simulink model "c960x4096_x14_7_r2013b_frb"  (R2013b)
settings: Solver=ode45  StartTime=0.0  StopTime=40960  RelTol=1e-3
undefined symbols (not defined in the file): sfp
libraries: xbsIndex_r4 x14620, casper_library_misc x61, dspsigops x32, casper_library_multipliers x24, simulink x18, xps_library x18
(part 11 of 79)

== system c960x4096_x14_7_r2013b_frb/p0_scale/SCALE_Re_&_Im_2 ==
  P_S : Inport
  SCALE : Inport  Port=2
  Convert : xbsIndex_r4/Convert  gui_display_data_type=Fixed-point  arith_type="Signed  (2's comp)"  n_bits=8  bin_pt=5  float_type=Single  exp_bits=8  fraction_bits=24  quantization=Truncate  overflow=Wrap  en=off  latency=0  dbl_ovrd=off  pipeline=off  block_type=convert
  Convert1 : xbsIndex_r4/Convert  gui_display_data_type=Fixed-point  arith_type="Signed  (2's comp)"  n_bits=8  bin_pt=5  float_type=Single  exp_bits=8  fraction_bits=24  quantization=Truncate  overflow=Wrap  en=off  latency=0  dbl_ovrd=off  pipeline=off  block_type=convert
  Mult : xbsIndex_r4/Mult  precision=Full  arith_type="Signed  (2's comp)"  n_bits=16  bin_pt=14  quantization=Truncate  overflow=Wrap  en=off  latency=4  dbl_ovrd=off  use_behavioral_HDL=off  opt=Speed  use_embedded=on  optimum_pipeline=off  pipeline=on  use_rpm=on  placement_style=Triangular  block_type=mult
  Mult1 : xbsIndex_r4/Mult  precision=Full  arith_type="Signed  (2's comp)"  n_bits=16  bin_pt=14  quantization=Truncate  overflow=Wrap  en=off  latency=4  dbl_ovrd=off  use_behavioral_HDL=off  opt=Speed  use_embedded=on  optimum_pipeline=off  pipeline=on  use_rpm=on  placement_style=Triangular  block_type=mult
  Reinterpret : xbsIndex_r4/Reinterpret  force_arith_type=on  arith_type="Signed  (2's comp)"  force_bin_pt=on  bin_pt=17  block_type=reinterpret
  Reinterpret1 : xbsIndex_r4/Reinterpret  force_arith_type=on  arith_type="Signed  (2's comp)"  force_bin_pt=on  bin_pt=17  block_type=reinterpret
  Slice : xbsIndex_r4/Slice  nbits=18  boolean_output=off  mode=Upper Bit Location + Width  bit1=0  base1=MSB of Input  bit0=0  base0=LSB of Input  dbl_ovrd=off  block_type=slice
  Slice1 : xbsIndex_r4/Slice  nbits=18  boolean_output=off  mode=Lower Bit Location + Width  bit1=0  base1=MSB of Input  bit0=0  base0=LSB of Input  dbl_ovrd=off  block_type=slice
  Re : Outport
  Im : Outport  Port=2
  wires:
  SCALE/1 -> Mult/2, Mult1/2
  P_S/1 -> Slice1/1, Slice/1
  Convert1/1 -> Im/1
  Convert/1 -> Re/1
  Mult1/1 -> Convert1/1
  Mult/1 -> Convert/1
  Reinterpret/1 -> Mult1/1
  Reinterpret1/1 -> Mult/1
  Slice1/1 -> Reinterpret/1
  Slice/1 -> Reinterpret1/1

== system c960x4096_x14_7_r2013b_frb/p0_scale/SCALE_Re_&_Im_3 ==
  P_S : Inport
  SCALE : Inport  Port=2
  Convert : xbsIndex_r4/Convert  gui_display_data_type=Fixed-point  arith_type="Signed  (2's comp)"  n_bits=8  bin_pt=5  float_type=Single  exp_bits=8  fraction_bits=24  quantization=Truncate  overflow=Wrap  en=off  latency=0  dbl_ovrd=off  pipeline=off  block_type=convert
  Convert1 : xbsIndex_r4/Convert  gui_display_data_type=Fixed-point  arith_type="Signed  (2's comp)"  n_bits=8  bin_pt=5  float_type=Single  exp_bits=8  fraction_bits=24  quantization=Truncate  overflow=Wrap  en=off  latency=0  dbl_ovrd=off  pipeline=off  block_type=convert
  Mult : xbsIndex_r4/Mult  precision=Full  arith_type="Signed  (2's comp)"  n_bits=16  bin_pt=14  quantization=Truncate  overflow=Wrap  en=off  latency=4  dbl_ovrd=off  use_behavioral_HDL=off  opt=Speed  use_embedded=on  optimum_pipeline=off  pipeline=on  use_rpm=on  placement_style=Triangular  block_type=mult
  Mult1 : xbsIndex_r4/Mult  precision=Full  arith_type="Signed  (2's comp)"  n_bits=16  bin_pt=14  quantization=Truncate  overflow=Wrap  en=off  latency=4  dbl_ovrd=off  use_behavioral_HDL=off  opt=Speed  use_embedded=on  optimum_pipeline=off  pipeline=on  use_rpm=on  placement_style=Triangular  block_type=mult
  Reinterpret : xbsIndex_r4/Reinterpret  force_arith_type=on  arith_type="Signed  (2's comp)"  force_bin_pt=on  bin_pt=17  block_type=reinterpret
  Reinterpret1 : xbsIndex_r4/Reinterpret  force_arith_type=on  arith_type="Signed  (2's comp)"  force_bin_pt=on  bin_pt=17  block_type=reinterpret
  Slice : xbsIndex_r4/Slice  nbits=18  boolean_output=off  mode=Upper Bit Location + Width  bit1=0  base1=MSB of Input  bit0=0  base0=LSB of Input  dbl_ovrd=off  block_type=slice
  Slice1 : xbsIndex_r4/Slice  nbits=18  boolean_output=off  mode=Lower Bit Location + Width  bit1=0  base1=MSB of Input  bit0=0  base0=LSB of Input  dbl_ovrd=off  block_type=slice
  Re : Outport
  Im : Outport  Port=2
  wires:
  SCALE/1 -> Mult/2, Mult1/2
  P_S/1 -> Slice1/1, Slice/1
  Convert1/1 -> Im/1
  Convert/1 -> Re/1
  Mult1/1 -> Convert1/1
  Mult/1 -> Convert/1
  Reinterpret/1 -> Mult1/1
  Reinterpret1/1 -> Mult/1
  Slice1/1 -> Reinterpret/1
  Slice/1 -> Reinterpret1/1

== system c960x4096_x14_7_r2013b_frb/p0_scale/SCALE_Re_&_Im_4 ==
  P_S : Inport
  SCALE : Inport  Port=2
  Convert : xbsIndex_r4/Convert  gui_display_data_type=Fixed-point  arith_type="Signed  (2's comp)"  n_bits=8  bin_pt=5  float_type=Single  exp_bits=8  fraction_bits=24  quantization=Truncate  overflow=Wrap  en=off  latency=0  dbl_ovrd=off  pipeline=off  block_type=convert
  Convert1 : xbsIndex_r4/Convert  gui_display_data_type=Fixed-point  arith_type="Signed  (2's comp)"  n_bits=8  bin_pt=5  float_type=Single  exp_bits=8  fraction_bits=24  quantization=Truncate  overflow=Wrap  en=off  latency=0  dbl_ovrd=off  pipeline=off  block_type=convert
  Mult : xbsIndex_r4/Mult  precision=Full  arith_type="Signed  (2's comp)"  n_bits=16  bin_pt=14  quantization=Truncate  overflow=Wrap  en=off  latency=4  dbl_ovrd=off  use_behavioral_HDL=off  opt=Speed  use_embedded=on  optimum_pipeline=off  pipeline=on  use_rpm=on  placement_style=Triangular  block_type=mult
  Mult1 : xbsIndex_r4/Mult  precision=Full  arith_type="Signed  (2's comp)"  n_bits=16  bin_pt=14  quantization=Truncate  overflow=Wrap  en=off  latency=4  dbl_ovrd=off  use_behavioral_HDL=off  opt=Speed  use_embedded=on  optimum_pipeline=off  pipeline=on  use_rpm=on  placement_style=Triangular  block_type=mult
  Reinterpret : xbsIndex_r4/Reinterpret  force_arith_type=on  arith_type="Signed  (2's comp)"  force_bin_pt=on  bin_pt=17  block_type=reinterpret
  Reinterpret1 : xbsIndex_r4/Reinterpret  force_arith_type=on  arith_type="Signed  (2's comp)"  force_bin_pt=on  bin_pt=17  block_type=reinterpret
  Slice : xbsIndex_r4/Slice  nbits=18  boolean_output=off  mode=Upper Bit Location + Width  bit1=0  base1=MSB of Input  bit0=0  base0=LSB of Input  dbl_ovrd=off  block_type=slice
  Slice1 : xbsIndex_r4/Slice  nbits=18  boolean_output=off  mode=Lower Bit Location + Width  bit1=0  base1=MSB of Input  bit0=0  base0=LSB of Input  dbl_ovrd=off  block_type=slice
  Re : Outport
  Im : Outport  Port=2
  wires:
  SCALE/1 -> Mult/2, Mult1/2
  P_S/1 -> Slice1/1, Slice/1
  Convert1/1 -> Im/1
  Convert/1 -> Re/1
  Mult1/1 -> Convert1/1
  Mult/1 -> Convert/1
  Reinterpret/1 -> Mult1/1
  Reinterpret1/1 -> Mult/1
  Slice1/1 -> Reinterpret/1
  Slice/1 -> Reinterpret1/1

== system c960x4096_x14_7_r2013b_frb/p0_scale/SCALE_Re_&_Im_5 ==
  P_S : Inport
  SCALE : Inport  Port=2
  Convert : xbsIndex_r4/Convert  gui_display_data_type=Fixed-point  arith_type="Signed  (2's comp)"  n_bits=8  bin_pt=5  float_type=Single  exp_bits=8  fraction_bits=24  quantization=Truncate  overflow=Wrap  en=off  latency=0  dbl_ovrd=off  pipeline=off  block_type=convert
  Convert1 : xbsIndex_r4/Convert  gui_display_data_type=Fixed-point  arith_type="Signed  (2's comp)"  n_bits=8  bin_pt=5  float_type=Single  exp_bits=8  fraction_bits=24  quantization=Truncate  overflow=Wrap  en=off  latency=0  dbl_ovrd=off  pipeline=off  block_type=convert
  Mult : xbsIndex_r4/Mult  precision=Full  arith_type="Signed  (2's comp)"  n_bits=16  bin_pt=14  quantization=Truncate  overflow=Wrap  en=off  latency=4  dbl_ovrd=off  use_behavioral_HDL=off  opt=Speed  use_embedded=on  optimum_pipeline=off  pipeline=on  use_rpm=on  placement_style=Triangular  block_type=mult
  Mult1 : xbsIndex_r4/Mult  precision=Full  arith_type="Signed  (2's comp)"  n_bits=16  bin_pt=14  quantization=Truncate  overflow=Wrap  en=off  latency=4  dbl_ovrd=off  use_behavioral_HDL=off  opt=Speed  use_embedded=on  optimum_pipeline=off  pipeline=on  use_rpm=on  placement_style=Triangular  block_type=mult
  Reinterpret : xbsIndex_r4/Reinterpret  force_arith_type=on  arith_type="Signed  (2's comp)"  force_bin_pt=on  bin_pt=17  block_type=reinterpret
  Reinterpret1 : xbsIndex_r4/Reinterpret  force_arith_type=on  arith_type="Signed  (2's comp)"  force_bin_pt=on  bin_pt=17  block_type=reinterpret
  Slice : xbsIndex_r4/Slice  nbits=18  boolean_output=off  mode=Upper Bit Location + Width  bit1=0  base1=MSB of Input  bit0=0  base0=LSB of Input  dbl_ovrd=off  block_type=slice
  Slice1 : xbsIndex_r4/Slice  nbits=18  boolean_output=off  mode=Lower Bit Location + Width  bit1=0  base1=MSB of Input  bit0=0  base0=LSB of Input  dbl_ovrd=off  block_type=slice
  Re : Outport
  Im : Outport  Port=2
  wires:
  SCALE/1 -> Mult/2, Mult1/2
  P_S/1 -> Slice1/1, Slice/1
  Convert1/1 -> Im/1
  Convert/1 -> Re/1
  Mult1/1 -> Convert1/1
  Mult/1 -> Convert/1
  Reinterpret/1 -> Mult1/1
  Reinterpret1/1 -> Mult/1
  Slice1/1 -> Reinterpret/1
  Slice/1 -> Reinterpret1/1

== system c960x4096_x14_7_r2013b_frb/p0_scale/SCALE_Re_&_Im_6 ==
  P_S : Inport
  SCALE : Inport  Port=2
  Convert : xbsIndex_r4/Convert  gui_display_data_type=Fixed-point  arith_type="Signed  (2's comp)"  n_bits=8  bin_pt=5  float_type=Single  exp_bits=8  fraction_bits=24  quantization=Truncate  overflow=Wrap  en=off  latency=0  dbl_ovrd=off  pipeline=off  block_type=convert
  Convert1 : xbsIndex_r4/Convert  gui_display_data_type=Fixed-point  arith_type="Signed  (2's comp)"  n_bits=8  bin_pt=5  float_type=Single  exp_bits=8  fraction_bits=24  quantization=Truncate  overflow=Wrap  en=off  latency=0  dbl_ovrd=off  pipeline=off  block_type=convert
  Mult : xbsIndex_r4/Mult  precision=Full  arith_type="Signed  (2's comp)"  n_bits=16  bin_pt=14  quantization=Truncate  overflow=Wrap  en=off  latency=4  dbl_ovrd=off  use_behavioral_HDL=off  opt=Speed  use_embedded=on  optimum_pipeline=off  pipeline=on  use_rpm=on  placement_style=Triangular  block_type=mult
  Mult1 : xbsIndex_r4/Mult  precision=Full  arith_type="Signed  (2's comp)"  n_bits=16  bin_pt=14  quantization=Truncate  overflow=Wrap  en=off  latency=4  dbl_ovrd=off  use_behavioral_HDL=off  opt=Speed  use_embedded=on  optimum_pipeline=off  pipeline=on  use_rpm=on  placement_style=Triangular  block_type=mult
  Reinterpret : xbsIndex_r4/Reinterpret  force_arith_type=on  arith_type="Signed  (2's comp)"  force_bin_pt=on  bin_pt=17  block_type=reinterpret
  Reinterpret1 : xbsIndex_r4/Reinterpret  force_arith_type=on  arith_type="Signed  (2's comp)"  force_bin_pt=on  bin_pt=17  block_type=reinterpret
  Slice : xbsIndex_r4/Slice  nbits=18  boolean_output=off  mode=Upper Bit Location + Width  bit1=0  base1=MSB of Input  bit0=0  base0=LSB of Input  dbl_ovrd=off  block_type=slice
  Slice1 : xbsIndex_r4/Slice  nbits=18  boolean_output=off  mode=Lower Bit Location + Width  bit1=0  base1=MSB of Input  bit0=0  base0=LSB of Input  dbl_ovrd=off  block_type=slice
  Re : Outport
  Im : Outport  Port=2
  wires:
  SCALE/1 -> Mult/2, Mult1/2
  P_S/1 -> Slice1/1, Slice/1
  Convert1/1 -> Im/1
  Convert/1 -> Re/1
  Mult1/1 -> Convert1/1
  Mult/1 -> Convert/1
  Reinterpret/1 -> Mult1/1
  Reinterpret1/1 -> Mult/1
  Slice1/1 -> Reinterpret/1
  Slice/1 -> Reinterpret1/1

== system c960x4096_x14_7_r2013b_frb/p0_scale/SCALE_Re_&_Im_7 ==
  P_S : Inport
  SCALE : Inport  Port=2
  Convert : xbsIndex_r4/Convert  gui_display_data_type=Fixed-point  arith_type="Signed  (2's comp)"  n_bits=8  bin_pt=5  float_type=Single  exp_bits=8  fraction_bits=24  quantization=Truncate  overflow=Wrap  en=off  latency=0  dbl_ovrd=off  pipeline=off  block_type=convert
  Convert1 : xbsIndex_r4/Convert  gui_display_data_type=Fixed-point  arith_type="Signed  (2's comp)"  n_bits=8  bin_pt=5  float_type=Single  exp_bits=8  fraction_bits=24  quantization=Truncate  overflow=Wrap  en=off  latency=0  dbl_ovrd=off  pipeline=off  block_type=convert
  Mult : xbsIndex_r4/Mult  precision=Full  arith_type="Signed  (2's comp)"  n_bits=16  bin_pt=14  quantization=Truncate  overflow=Wrap  en=off  latency=4  dbl_ovrd=off  use_behavioral_HDL=off  opt=Speed  use_embedded=on  optimum_pipeline=off  pipeline=on  use_rpm=on  placement_style=Triangular  block_type=mult
  Mult1 : xbsIndex_r4/Mult  precision=Full  arith_type="Signed  (2's comp)"  n_bits=16  bin_pt=14  quantization=Truncate  overflow=Wrap  en=off  latency=4  dbl_ovrd=off  use_behavioral_HDL=off  opt=Speed  use_embedded=on  optimum_pipeline=off  pipeline=on  use_rpm=on  placement_style=Triangular  block_type=mult
  Reinterpret : xbsIndex_r4/Reinterpret  force_arith_type=on  arith_type="Signed  (2's comp)"  force_bin_pt=on  bin_pt=17  block_type=reinterpret
  Reinterpret1 : xbsIndex_r4/Reinterpret  force_arith_type=on  arith_type="Signed  (2's comp)"  force_bin_pt=on  bin_pt=17  block_type=reinterpret
  Slice : xbsIndex_r4/Slice  nbits=18  boolean_output=off  mode=Upper Bit Location + Width  bit1=0  base1=MSB of Input  bit0=0  base0=LSB of Input  dbl_ovrd=off  block_type=slice
  Slice1 : xbsIndex_r4/Slice  nbits=18  boolean_output=off  mode=Lower Bit Location + Width  bit1=0  base1=MSB of Input  bit0=0  base0=LSB of Input  dbl_ovrd=off  block_type=slice
  Re : Outport
  Im : Outport  Port=2
  wires:
  SCALE/1 -> Mult/2, Mult1/2
  P_S/1 -> Slice1/1, Slice/1
  Convert1/1 -> Im/1
  Convert/1 -> Re/1
  Mult1/1 -> Convert1/1
  Mult/1 -> Convert/1
  Reinterpret/1 -> Mult1/1
  Reinterpret1/1 -> Mult/1
  Slice1/1 -> Reinterpret/1
  Slice/1 -> Reinterpret1/1

== system c960x4096_x14_7_r2013b_frb/p1_adc/Subsystem1 ==
  In1 : Inport
  In2 : Inport  Port=2
  In3 : Inport  Port=3
  In4 : Inport  Port=4
  In5 : Inport  Port=5
  In6 : Inport  Port=6
  In7 : Inport  Port=7
  In8 : Inport  Port=8
  In9 : Inport  Port=9
  In10 : Inport  Port=10
  In11 : Inport  Port=11
  In12 : Inport  Port=12
  In13 : Inport  Port=13
  In14 : Inport  Port=14
  In15 : Inport  Port=15
  In16 : Inport  Port=16
  Delay{1..10,18..20,22..24} (16 alike) : xbsIndex_r4/Delay  rst=off  infoeditControl=Selection of Reset will increase slice count due to use of real FFs and instead of SRLs  en=off  latency=1  dbl_ovrd=off  reg_retiming=on  block_type=delay
      settings: block_version=11.4
  DocBlock : simulink/Model-Wide Utilities/DocBlock  DocumentType=Text
      content=|
      | - JMR, 04/30/13
      | Converter blocks needed to convert the ASIAA ADC output from offset
      | notation (0 - 255 corresponds to -full scale to +full scale) to 2's
      | complement (-128 to +127).  Per email from Glenn Jones, 04/17/13
  bus_create : Subsystem  AncestorBlock=casper_library_flow_control/bus_create  mask(bus_create){inputNum=16}
      mask prompts: inputNum "Number of inputs:"
      mask init:
      | bus_create_init(gcb,...
      |     'inputNum', inputNum);
  converter : Subsystem
  converter1 : Subsystem
  converter10 : Subsystem
  converter11 : Subsystem
  converter12 : Subsystem
  converter13 : Subsystem
  converter14 : Subsystem
  converter15 : Subsystem
  converter2 : Subsystem
  converter3 : Subsystem
  converter4 : Subsystem
  converter5 : Subsystem
  converter6 : Subsystem
  converter7 : Subsystem
  converter8 : Subsystem
  converter9 : Subsystem
  Out1 : Outport
  wires:
  Delay6/1 -> bus_create/16(in16)
  Delay5/1 -> bus_create/15(in15)
  Delay4/1 -> bus_create/14(in14)
  Delay3/1 -> bus_create/13(in13)
  Delay2/1 -> bus_create/12(in12)
  Delay1/1 -> bus_create/11(in11)
  Delay10/1 -> bus_create/10(in10)
  Delay8/1 -> bus_create/9(in9)
  Delay24/1 -> bus_create/8(in8)
  Delay23/1 -> bus_create/7(in7)
  Delay22/1 -> bus_create/6(in6)
  Delay20/1 -> bus_create/5(in5)
  Delay19/1 -> bus_create/4(in4)
  Delay18/1 -> bus_create/3(in3)
  Delay9/1 -> bus_create/2(in2)
  Delay7/1 -> bus_create/1(in1)
  converter7/1(s8_7) -> Delay24/1
  converter6/1(s8_7) -> Delay23/1
  converter5/1(s8_7) -> Delay22/1
  converter4/1(s8_7) -> Delay20/1
  converter3/1(s8_7) -> Delay19/1
  converter2/1(s8_7) -> Delay18/1
  converter1/1(s8_7) -> Delay9/1
  converter/1(s8_7) -> Delay7/1
  converter8/1(s8_7) -> Delay8/1
  converter9/1(s8_7) -> Delay10/1
  converter10/1(s8_7) -> Delay1/1
  converter11/1(s8_7) -> Delay2/1
  converter12/1(s8_7) -> Delay3/1
  converter13/1(s8_7) -> Delay4/1
  converter14/1(s8_7) -> Delay5/1
  converter15/1(s8_7) -> Delay6/1
  In16/1 -> converter15/1(u8_0)
  In15/1 -> converter14/1(u8_0)
  In14/1 -> converter13/1(u8_0)
  In13/1 -> converter12/1(u8_0)
  In12/1 -> converter11/1(u8_0)
  In11/1 -> converter10/1(u8_0)
  In10/1 -> converter9/1(u8_0)
  In9/1 -> converter8/1(u8_0)
  In8/1 -> converter7/1(u8_0)
  In7/1 -> converter6/1(u8_0)
  In6/1 -> converter5/1(u8_0)
  In5/1 -> converter4/1(u8_0)
  In4/1 -> converter3/1(u8_0)
  In3/1 -> converter2/1(u8_0)
  In2/1 -> converter1/1(u8_0)
  In1/1 -> converter/1(u8_0)
  bus_create/1(bus_out) -> Out1/1

== system c960x4096_x14_7_r2013b_frb/p1_adc/asiaa_adc5g1 ==
  sim_a : Inport
  sim_sync : Inport  Port=2
  bias_a : Bias  Bias=128  SaturateOnIntegerOverflow=on
  c960x4096_x14_7_frbout_p1_adc_asiaa_adc5g1_sync : xbsIndex_r4/Gateway In  gui_display_data_type=Fixed-point  arith_type=Boolean  n_bits=16  bin_pt=14  preci_type=Single  exp_width=8  frac_width=24  quantization="Round  (unbiased: +/- Inf)"  overflow=Saturate  period=1  dbl_ovrd=off  timing_constraint=None  locs_specified=off  LOCs={}  UseAsADC=off  ADCChannel='1'  inherit_from_input=off  hdl_port=on  block_type=gatewayin
  c960x4096_x14_7_frbout_p1_adc_asiaa_adc5g1_user_data_i{0..7} (8 alike) : xbsIndex_r4/Gateway In  gui_display_data_type=Fixed-point  arith_type=Unsigned  n_bits=8  bin_pt=0  preci_type=Single  exp_width=8  frac_width=24  quantization=Truncate  overflow=Wrap  period=1  dbl_ovrd=off  timing_constraint=None  locs_specified=off  LOCs={}  UseAsADC=off  ADCChannel='1'  inherit_from_input=off  hdl_port=on  block_type=gatewayin
  c960x4096_x14_7_frbout_p1_adc_asiaa_adc5g1_user_data_q{0..7} (8 alike) : xbsIndex_r4/Gateway In  gui_display_data_type=Fixed-point  arith_type=Unsigned  n_bits=8  bin_pt=0  preci_type=Single  exp_width=8  frac_width=24  quantization=Truncate  overflow=Wrap  period=1  dbl_ovrd=off  timing_constraint=None  locs_specified=off  LOCs={}  UseAsADC=off  ADCChannel='1'  inherit_from_input=off  hdl_port=on  block_type=gatewayin
  delay_a0 : Delay  InitialCondition=0  InputProcessing=Inherited
  delay_a{1..15} (15 alike) : Delay  DelayLength=1  InitialCondition=0  InputProcessing=Inherited
  downsample_a0 : dspsigops/Downsample  N=16  phase=0  RateOptions=Allow multirate processing  smode=Allow multirate  fmode=Maintain input frame size  ic=0
  downsample_a1 : dspsigops/Downsample  N=16  phase=1  RateOptions=Allow multirate processing  smode=Allow multirate  fmode=Maintain input frame size  ic=0
  downsample_a10 : dspsigops/Downsample  N=16  phase=10  RateOptions=Allow multirate processing  smode=Allow multirate  fmode=Maintain input frame size  ic=0
  downsample_a11 : dspsigops/Downsample  N=16  phase=11  RateOptions=Allow multirate processing  smode=Allow multirate  fmode=Maintain input frame size  ic=0
  downsample_a12 : dspsigops/Downsample  N=16  phase=12  RateOptions=Allow multirate processing  smode=Allow multirate  fmode=Maintain input frame size  ic=0
  downsample_a13 : dspsigops/Downsample  N=16  phase=13  RateOptions=Allow multirate processing  smode=Allow multirate  fmode=Maintain input frame size  ic=0
  downsample_a14 : dspsigops/Downsample  N=16  phase=14  RateOptions=Allow multirate processing  smode=Allow multirate  fmode=Maintain input frame size  ic=0
  downsample_a15 : dspsigops/Downsample  N=16  phase=15  RateOptions=Allow multirate processing  smode=Allow multirate  fmode=Maintain input frame size  ic=0
  downsample_a2 : dspsigops/Downsample  N=16  phase=2  RateOptions=Allow multirate processing  smode=Allow multirate  fmode=Maintain input frame size  ic=0
  downsample_a3 : dspsigops/Downsample  N=16  phase=3  RateOptions=Allow multirate processing  smode=Allow multirate  fmode=Maintain input frame size  ic=0
  downsample_a4 : dspsigops/Downsample  N=16  phase=4  RateOptions=Allow multirate processing  smode=Allow multirate  fmode=Maintain input frame size  ic=0
  downsample_a5 : dspsigops/Downsample  N=16  phase=5  RateOptions=Allow multirate processing  smode=Allow multirate  fmode=Maintain input frame size  ic=0
  downsample_a6 : dspsigops/Downsample  N=16  phase=6  RateOptions=Allow multirate processing  smode=Allow multirate  fmode=Maintain input frame size  ic=0
  downsample_a7 : dspsigops/Downsample  N=16  phase=7  RateOptions=Allow multirate processing  smode=Allow multirate  fmode=Maintain input frame size  ic=0
  downsample_a8 : dspsigops/Downsample  N=16  phase=8  RateOptions=Allow multirate processing  smode=Allow multirate  fmode=Maintain input frame size  ic=0
  downsample_a9 : dspsigops/Downsample  N=16  phase=9  RateOptions=Allow multirate processing  smode=Allow multirate  fmode=Maintain input frame size  ic=0
  gain_a : Gain  Gain=128  SaturateOnIntegerOverflow=on  OutDataTypeStr=Inherit: Same as input  ParamDataTypeStr=Inherit: Same as input
  a0 : Outport
  a1 : Outport  Port=2
  a2 : Outport  Port=3
  a3 : Outport  Port=4
  a4 : Outport  Port=5
  a5 : Outport  Port=6
  a6 : Outport  Port=7
  a7 : Outport  Port=8
  a8 : Outport  Port=9
  a9 : Outport  Port=10
  a10 : Outport  Port=11
  a11 : Outport  Port=12
  a12 : Outport  Port=13
  a13 : Outport  Port=14
  a14 : Outport  Port=15
  a15 : Outport  Port=16
  sync_out : Outport  Port=17
  wires:
  sim_a/1 -> gain_a/1
  gain_a/1 -> bias_a/1
  bias_a/1 -> downsample_a0/1, downsample_a1/1, downsample_a2/1, downsample_a3/1, downsample_a4/1, downsample_a5/1, downsample_a6/1, downsample_a7/1, downsample_a8/1, downsample_a9/1, downsample_a10/1, downsample_a11/1, downsample_a12/1, downsample_a13/1, downsample_a14/1, downsample_a15/1
  downsample_a0/1 -> delay_a0/1
  delay_a0/1 -> c960x4096_x14_7_frbout_p1_adc_asiaa_adc5g1_user_data_i0/1
  c960x4096_x14_7_frbout_p1_adc_asiaa_adc5g1_user_data_i0/1 -> a0/1
  downsample_a1/1 -> delay_a1/1
  delay_a1/1 -> c960x4096_x14_7_frbout_p1_adc_asiaa_adc5g1_user_data_i1/1
  c960x4096_x14_7_frbout_p1_adc_asiaa_adc5g1_user_data_i1/1 -> a1/1
  downsample_a2/1 -> delay_a2/1
  delay_a2/1 -> c960x4096_x14_7_frbout_p1_adc_asiaa_adc5g1_user_data_i2/1
  c960x4096_x14_7_frbout_p1_adc_asiaa_adc5g1_user_data_i2/1 -> a2/1
  downsample_a3/1 -> delay_a3/1
  delay_a3/1 -> c960x4096_x14_7_frbout_p1_adc_asiaa_adc5g1_user_data_i3/1
  c960x4096_x14_7_frbout_p1_adc_asiaa_adc5g1_user_data_i3/1 -> a3/1
  downsample_a4/1 -> delay_a4/1
  delay_a4/1 -> c960x4096_x14_7_frbout_p1_adc_asiaa_adc5g1_user_data_i4/1
  c960x4096_x14_7_frbout_p1_adc_asiaa_adc5g1_user_data_i4/1 -> a4/1
  downsample_a5/1 -> delay_a5/1
  delay_a5/1 -> c960x4096_x14_7_frbout_p1_adc_asiaa_adc5g1_user_data_i5/1
  c960x4096_x14_7_frbout_p1_adc_asiaa_adc5g1_user_data_i5/1 -> a5/1
  downsample_a6/1 -> delay_a6/1
  delay_a6/1 -> c960x4096_x14_7_frbout_p1_adc_asiaa_adc5g1_user_data_i6/1
  c960x4096_x14_7_frbout_p1_adc_asiaa_adc5g1_user_data_i6/1 -> a6/1
  downsample_a7/1 -> delay_a7/1
  delay_a7/1 -> c960x4096_x14_7_frbout_p1_adc_asiaa_adc5g1_user_data_i7/1
  c960x4096_x14_7_frbout_p1_adc_asiaa_adc5g1_user_data_i7/1 -> a7/1
  downsample_a8/1 -> delay_a8/1
  delay_a8/1 -> c960x4096_x14_7_frbout_p1_adc_asiaa_adc5g1_user_data_q0/1
  c960x4096_x14_7_frbout_p1_adc_asiaa_adc5g1_user_data_q0/1 -> a8/1
  downsample_a9/1 -> delay_a9/1
  delay_a9/1 -> c960x4096_x14_7_frbout_p1_adc_asiaa_adc5g1_user_data_q1/1
  c960x4096_x14_7_frbout_p1_adc_asiaa_adc5g1_user_data_q1/1 -> a9/1
  downsample_a10/1 -> delay_a10/1
  delay_a10/1 -> c960x4096_x14_7_frbout_p1_adc_asiaa_adc5g1_user_data_q2/1
  c960x4096_x14_7_frbout_p1_adc_asiaa_adc5g1_user_data_q2/1 -> a10/1
  downsample_a11/1 -> delay_a11/1
  delay_a11/1 -> c960x4096_x14_7_frbout_p1_adc_asiaa_adc5g1_user_data_q3/1
  c960x4096_x14_7_frbout_p1_adc_asiaa_adc5g1_user_data_q3/1 -> a11/1
  downsample_a12/1 -> delay_a12/1
  delay_a12/1 -> c960x4096_x14_7_frbout_p1_adc_asiaa_adc5g1_user_data_q4/1
  c960x4096_x14_7_frbout_p1_adc_asiaa_adc5g1_user_data_q4/1 -> a12/1
  downsample_a13/1 -> delay_a13/1
  delay_a13/1 -> c960x4096_x14_7_frbout_p1_adc_asiaa_adc5g1_user_data_q5/1
  c960x4096_x14_7_frbout_p1_adc_asiaa_adc5g1_user_data_q5/1 -> a13/1
  downsample_a14/1 -> delay_a14/1
  delay_a14/1 -> c960x4096_x14_7_frbout_p1_adc_asiaa_adc5g1_user_data_q6/1
  c960x4096_x14_7_frbout_p1_adc_asiaa_adc5g1_user_data_q6/1 -> a14/1
  downsample_a15/1 -> delay_a15/1
  delay_a15/1 -> c960x4096_x14_7_frbout_p1_adc_asiaa_adc5g1_user_data_q7/1
  c960x4096_x14_7_frbout_p1_adc_asiaa_adc5g1_user_data_q7/1 -> a15/1
  sim_sync/1 -> c960x4096_x14_7_frbout_p1_adc_asiaa_adc5g1_sync/1
  c960x4096_x14_7_frbout_p1_adc_asiaa_adc5g1_sync/1 -> sync_out/1

== system c960x4096_x14_7_r2013b_frb/p1_scale/SCALE_Re_&_Im_0 ==
  P_S : Inport
  SCALE : Inport  Port=2
  Convert : xbsIndex_r4/Convert  gui_display_data_type=Fixed-point  arith_type="Signed  (2's comp)"  n_bits=8  bin_pt=5  float_type=Single  exp_bits=8  fraction_bits=24  quantization=Truncate  overflow=Wrap  en=off  latency=0  dbl_ovrd=off  pipeline=off  block_type=convert
  Convert1 : xbsIndex_r4/Convert  gui_display_data_type=Fixed-point  arith_type="Signed  (2's comp)"  n_bits=8  bin_pt=5  float_type=Single  exp_bits=8  fraction_bits=24  quantization=Truncate  overflow=Wrap  en=off  latency=0  dbl_ovrd=off  pipeline=off  block_type=convert
  Mult : xbsIndex_r4/Mult  precision=Full  arith_type="Signed  (2's comp)"  n_bits=16  bin_pt=14  quantization=Truncate  overflow=Wrap  en=off  latency=4  dbl_ovrd=off  use_behavioral_HDL=off  opt=Speed  use_embedded=on  optimum_pipeline=off  pipeline=on  use_rpm=on  placement_style=Triangular  block_type=mult
  Mult1 : xbsIndex_r4/Mult  precision=Full  arith_type="Signed  (2's comp)"  n_bits=16  bin_pt=14  quantization=Truncate  overflow=Wrap  en=off  latency=4  dbl_ovrd=off  use_behavioral_HDL=off  opt=Speed  use_embedded=on  optimum_pipeline=off  pipeline=on  use_rpm=on  placement_style=Triangular  block_type=mult
  Reinterpret : xbsIndex_r4/Reinterpret  force_arith_type=on  arith_type="Signed  (2's comp)"  force_bin_pt=on  bin_pt=17  block_type=reinterpret
  Reinterpret1 : xbsIndex_r4/Reinterpret  force_arith_type=on  arith_type="Signed  (2's comp)"  force_bin_pt=on  bin_pt=17  block_type=reinterpret
  Slice : xbsIndex_r4/Slice  nbits=18  boolean_output=off  mode=Upper Bit Location + Width  bit1=0  base1=MSB of Input  bit0=0  base0=LSB of Input  dbl_ovrd=off  block_type=slice
  Slice1 : xbsIndex_r4/Slice  nbits=18  boolean_output=off  mode=Lower Bit Location + Width  bit1=0  base1=MSB of Input  bit0=0  base0=LSB of Input  dbl_ovrd=off  block_type=slice
  Re : Outport
  Im : Outport  Port=2
  wires:
  SCALE/1 -> Mult/2, Mult1/2
  P_S/1 -> Slice1/1, Slice/1
  Convert1/1 -> Im/1
  Convert/1 -> Re/1
  Mult1/1 -> Convert1/1
  Mult/1 -> Convert/1
  Reinterpret/1 -> Mult1/1
  Reinterpret1/1 -> Mult/1
  Slice1/1 -> Reinterpret/1
  Slice/1 -> Reinterpret1/1

== system c960x4096_x14_7_r2013b_frb/p1_scale/SCALE_Re_&_Im_1 ==
  P_S : Inport
  SCALE : Inport  Port=2
  Convert : xbsIndex_r4/Convert  gui_display_data_type=Fixed-point  arith_type="Signed  (2's comp)"  n_bits=8  bin_pt=5  float_type=Single  exp_bits=8  fraction_bits=24  quantization=Truncate  overflow=Wrap  en=off  latency=0  dbl_ovrd=off  pipeline=off  block_type=convert
  Convert1 : xbsIndex_r4/Convert  gui_display_data_type=Fixed-point  arith_type="Signed  (2's comp)"  n_bits=8  bin_pt=5  float_type=Single  exp_bits=8  fraction_bits=24  quantization=Truncate  overflow=Wrap  en=off  latency=0  dbl_ovrd=off  pipeline=off  block_type=convert
  Mult : xbsIndex_r4/Mult  precision=Full  arith_type="Signed  (2's comp)"  n_bits=16  bin_pt=14  quantization=Truncate  overflow=Wrap  en=off  latency=4  dbl_ovrd=off  use_behavioral_HDL=off  opt=Speed  use_embedded=on  optimum_pipeline=off  pipeline=on  use_rpm=on  placement_style=Triangular  block_type=mult
  Mult1 : xbsIndex_r4/Mult  precision=Full  arith_type="Signed  (2's comp)"  n_bits=16  bin_pt=14  quantization=Truncate  overflow=Wrap  en=off  latency=4  dbl_ovrd=off  use_behavioral_HDL=off  opt=Speed  use_embedded=on  optimum_pipeline=off  pipeline=on  use_rpm=on  placement_style=Triangular  block_type=mult
  Reinterpret : xbsIndex_r4/Reinterpret  force_arith_type=on  arith_type="Signed  (2's comp)"  force_bin_pt=on  bin_pt=17  block_type=reinterpret
  Reinterpret1 : xbsIndex_r4/Reinterpret  force_arith_type=on  arith_type="Signed  (2's comp)"  force_bin_pt=on  bin_pt=17  block_type=reinterpret
  Slice : xbsIndex_r4/Slice  nbits=18  boolean_output=off  mode=Upper Bit Location + Width  bit1=0  base1=MSB of Input  bit0=0  base0=LSB of Input  dbl_ovrd=off  block_type=slice
  Slice1 : xbsIndex_r4/Slice  nbits=18  boolean_output=off  mode=Lower Bit Location + Width  bit1=0  base1=MSB of Input  bit0=0  base0=LSB of Input  dbl_ovrd=off  block_type=slice
  Re : Outport
  Im : Outport  Port=2
  wires:
  SCALE/1 -> Mult/2, Mult1/2
  P_S/1 -> Slice1/1, Slice/1
  Convert1/1 -> Im/1
  Convert/1 -> Re/1
  Mult1/1 -> Convert1/1
  Mult/1 -> Convert/1
  Reinterpret/1 -> Mult1/1
  Reinterpret1/1 -> Mult/1
  Slice1/1 -> Reinterpret/1
  Slice/1 -> Reinterpret1/1

== system c960x4096_x14_7_r2013b_frb/p1_scale/SCALE_Re_&_Im_2 ==
  P_S : Inport
  SCALE : Inport  Port=2
  Convert : xbsIndex_r4/Convert  gui_display_data_type=Fixed-point  arith_type="Signed  (2's comp)"  n_bits=8  bin_pt=5  float_type=Single  exp_bits=8  fraction_bits=24  quantization=Truncate  overflow=Wrap  en=off  latency=0  dbl_ovrd=off  pipeline=off  block_type=convert
  Convert1 : xbsIndex_r4/Convert  gui_display_data_type=Fixed-point  arith_type="Signed  (2's comp)"  n_bits=8  bin_pt=5  float_type=Single  exp_bits=8  fraction_bits=24  quantization=Truncate  overflow=Wrap  en=off  latency=0  dbl_ovrd=off  pipeline=off  block_type=convert
  Mult : xbsIndex_r4/Mult  precision=Full  arith_type="Signed  (2's comp)"  n_bits=16  bin_pt=14  quantization=Truncate  overflow=Wrap  en=off  latency=4  dbl_ovrd=off  use_behavioral_HDL=off  opt=Speed  use_embedded=on  optimum_pipeline=off  pipeline=on  use_rpm=on  placement_style=Triangular  block_type=mult
  Mult1 : xbsIndex_r4/Mult  precision=Full  arith_type="Signed  (2's comp)"  n_bits=16  bin_pt=14  quantization=Truncate  overflow=Wrap  en=off  latency=4  dbl_ovrd=off  use_behavioral_HDL=off  opt=Speed  use_embedded=on  optimum_pipeline=off  pipeline=on  use_rpm=on  placement_style=Triangular  block_type=mult
  Reinterpret : xbsIndex_r4/Reinterpret  force_arith_type=on  arith_type="Signed  (2's comp)"  force_bin_pt=on  bin_pt=17  block_type=reinterpret
  Reinterpret1 : xbsIndex_r4/Reinterpret  force_arith_type=on  arith_type="Signed  (2's comp)"  force_bin_pt=on  bin_pt=17  block_type=reinterpret
  Slice : xbsIndex_r4/Slice  nbits=18  boolean_output=off  mode=Upper Bit Location + Width  bit1=0  base1=MSB of Input  bit0=0  base0=LSB of Input  dbl_ovrd=off  block_type=slice
  Slice1 : xbsIndex_r4/Slice  nbits=18  boolean_output=off  mode=Lower Bit Location + Width  bit1=0  base1=MSB of Input  bit0=0  base0=LSB of Input  dbl_ovrd=off  block_type=slice
  Re : Outport
  Im : Outport  Port=2
  wires:
  SCALE/1 -> Mult/2, Mult1/2
  P_S/1 -> Slice1/1, Slice/1
  Convert1/1 -> Im/1
  Convert/1 -> Re/1
  Mult1/1 -> Convert1/1
  Mult/1 -> Convert/1
  Reinterpret/1 -> Mult1/1
  Reinterpret1/1 -> Mult/1
  Slice1/1 -> Reinterpret/1
  Slice/1 -> Reinterpret1/1

== system c960x4096_x14_7_r2013b_frb/p1_scale/SCALE_Re_&_Im_3 ==
  P_S : Inport
  SCALE : Inport  Port=2
  Convert : xbsIndex_r4/Convert  gui_display_data_type=Fixed-point  arith_type="Signed  (2's comp)"  n_bits=8  bin_pt=5  float_type=Single  exp_bits=8  fraction_bits=24  quantization=Truncate  overflow=Wrap  en=off  latency=0  dbl_ovrd=off  pipeline=off  block_type=convert
  Convert1 : xbsIndex_r4/Convert  gui_display_data_type=Fixed-point  arith_type="Signed  (2's comp)"  n_bits=8  bin_pt=5  float_type=Single  exp_bits=8  fraction_bits=24  quantization=Truncate  overflow=Wrap  en=off  latency=0  dbl_ovrd=off  pipeline=off  block_type=convert
  Mult : xbsIndex_r4/Mult  precision=Full  arith_type="Signed  (2's comp)"  n_bits=16  bin_pt=14  quantization=Truncate  overflow=Wrap  en=off  latency=4  dbl_ovrd=off  use_behavioral_HDL=off  opt=Speed  use_embedded=on  optimum_pipeline=off  pipeline=on  use_rpm=on  placement_style=Triangular  block_type=mult
  Mult1 : xbsIndex_r4/Mult  precision=Full  arith_type="Signed  (2's comp)"  n_bits=16  bin_pt=14  quantization=Truncate  overflow=Wrap  en=off  latency=4  dbl_ovrd=off  use_behavioral_HDL=off  opt=Speed  use_embedded=on  optimum_pipeline=off  pipeline=on  use_rpm=on  placement_style=Triangular  block_type=mult
  Reinterpret : xbsIndex_r4/Reinterpret  force_arith_type=on  arith_type="Signed  (2's comp)"  force_bin_pt=on  bin_pt=17  block_type=reinterpret
  Reinterpret1 : xbsIndex_r4/Reinterpret  force_arith_type=on  arith_type="Signed  (2's comp)"  force_bin_pt=on  bin_pt=17  block_type=reinterpret
  Slice : xbsIndex_r4/Slice  nbits=18  boolean_output=off  mode=Upper Bit Location + Width  bit1=0  base1=MSB of Input  bit0=0  base0=LSB of Input  dbl_ovrd=off  block_type=slice
  Slice1 : xbsIndex_r4/Slice  nbits=18  boolean_output=off  mode=Lower Bit Location + Width  bit1=0  base1=MSB of Input  bit0=0  base0=LSB of Input  dbl_ovrd=off  block_type=slice
  Re : Outport
  Im : Outport  Port=2
  wires:
  SCALE/1 -> Mult/2, Mult1/2
  P_S/1 -> Slice1/1, Slice/1
  Convert1/1 -> Im/1
  Convert/1 -> Re/1
  Mult1/1 -> Convert1/1
  Mult/1 -> Convert/1
  Reinterpret/1 -> Mult1/1
  Reinterpret1/1 -> Mult/1
  Slice1/1 -> Reinterpret/1
  Slice/1 -> Reinterpret1/1

== system c960x4096_x14_7_r2013b_frb/p1_scale/SCALE_Re_&_Im_4 ==
  P_S : Inport
  SCALE : Inport  Port=2
  Convert : xbsIndex_r4/Convert  gui_display_data_type=Fixed-point  arith_type="Signed  (2's comp)"  n_bits=8  bin_pt=5  float_type=Single  exp_bits=8  fraction_bits=24  quantization=Truncate  overflow=Wrap  en=off  latency=0  dbl_ovrd=off  pipeline=off  block_type=convert
  Convert1 : xbsIndex_r4/Convert  gui_display_data_type=Fixed-point  arith_type="Signed  (2's comp)"  n_bits=8  bin_pt=5  float_type=Single  exp_bits=8  fraction_bits=24  quantization=Truncate  overflow=Wrap  en=off  latency=0  dbl_ovrd=off  pipeline=off  block_type=convert
  Mult : xbsIndex_r4/Mult  precision=Full  arith_type="Signed  (2's comp)"  n_bits=16  bin_pt=14  quantization=Truncate  overflow=Wrap  en=off  latency=4  dbl_ovrd=off  use_behavioral_HDL=off  opt=Speed  use_embedded=on  optimum_pipeline=off  pipeline=on  use_rpm=on  placement_style=Triangular  block_type=mult
  Mult1 : xbsIndex_r4/Mult  precision=Full  arith_type="Signed  (2's comp)"  n_bits=16  bin_pt=14  quantization=Truncate  overflow=Wrap  en=off  latency=4  dbl_ovrd=off  use_behavioral_HDL=off  opt=Speed  use_embedded=on  optimum_pipeline=off  pipeline=on  use_rpm=on  placement_style=Triangular  block_type=mult
  Reinterpret : xbsIndex_r4/Reinterpret  force_arith_type=on  arith_type="Signed  (2's comp)"  force_bin_pt=on  bin_pt=17  block_type=reinterpret
  Reinterpret1 : xbsIndex_r4/Reinterpret  force_arith_type=on  arith_type="Signed  (2's comp)"  force_bin_pt=on  bin_pt=17  block_type=reinterpret
  Slice : xbsIndex_r4/Slice  nbits=18  boolean_output=off  mode=Upper Bit Location + Width  bit1=0  base1=MSB of Input  bit0=0  base0=LSB of Input  dbl_ovrd=off  block_type=slice
  Slice1 : xbsIndex_r4/Slice  nbits=18  boolean_output=off  mode=Lower Bit Location + Width  bit1=0  base1=MSB of Input  bit0=0  base0=LSB of Input  dbl_ovrd=off  block_type=slice
  Re : Outport
  Im : Outport  Port=2
  wires:
  SCALE/1 -> Mult/2, Mult1/2
  P_S/1 -> Slice1/1, Slice/1
  Convert1/1 -> Im/1
  Convert/1 -> Re/1
  Mult1/1 -> Convert1/1
  Mult/1 -> Convert/1
  Reinterpret/1 -> Mult1/1
  Reinterpret1/1 -> Mult/1
  Slice1/1 -> Reinterpret/1
  Slice/1 -> Reinterpret1/1

== system c960x4096_x14_7_r2013b_frb/p1_scale/SCALE_Re_&_Im_5 ==
  P_S : Inport
  SCALE : Inport  Port=2
  Convert : xbsIndex_r4/Convert  gui_display_data_type=Fixed-point  arith_type="Signed  (2's comp)"  n_bits=8  bin_pt=5  float_type=Single  exp_bits=8  fraction_bits=24  quantization=Truncate  overflow=Wrap  en=off  latency=0  dbl_ovrd=off  pipeline=off  block_type=convert
  Convert1 : xbsIndex_r4/Convert  gui_display_data_type=Fixed-point  arith_type="Signed  (2's comp)"  n_bits=8  bin_pt=5  float_type=Single  exp_bits=8  fraction_bits=24  quantization=Truncate  overflow=Wrap  en=off  latency=0  dbl_ovrd=off  pipeline=off  block_type=convert
  Mult : xbsIndex_r4/Mult  precision=Full  arith_type="Signed  (2's comp)"  n_bits=16  bin_pt=14  quantization=Truncate  overflow=Wrap  en=off  latency=4  dbl_ovrd=off  use_behavioral_HDL=off  opt=Speed  use_embedded=on  optimum_pipeline=off  pipeline=on  use_rpm=on  placement_style=Triangular  block_type=mult
  Mult1 : xbsIndex_r4/Mult  precision=Full  arith_type="Signed  (2's comp)"  n_bits=16  bin_pt=14  quantization=Truncate  overflow=Wrap  en=off  latency=4  dbl_ovrd=off  use_behavioral_HDL=off  opt=Speed  use_embedded=on  optimum_pipeline=off  pipeline=on  use_rpm=on  placement_style=Triangular  block_type=mult
  Reinterpret : xbsIndex_r4/Reinterpret  force_arith_type=on  arith_type="Signed  (2's comp)"  force_bin_pt=on  bin_pt=17  block_type=reinterpret
  Reinterpret1 : xbsIndex_r4/Reinterpret  force_arith_type=on  arith_type="Signed  (2's comp)"  force_bin_pt=on  bin_pt=17  block_type=reinterpret
  Slice : xbsIndex_r4/Slice  nbits=18  boolean_output=off  mode=Upper Bit Location + Width  bit1=0  base1=MSB of Input  bit0=0  base0=LSB of Input  dbl_ovrd=off  block_type=slice
  Slice1 : xbsIndex_r4/Slice  nbits=18  boolean_output=off  mode=Lower Bit Location + Width  bit1=0  base1=MSB of Input  bit0=0  base0=LSB of Input  dbl_ovrd=off  block_type=slice
  Re : Outport
  Im : Outport  Port=2
  wires:
  SCALE/1 -> Mult/2, Mult1/2
  P_S/1 -> Slice1/1, Slice/1
  Convert1/1 -> Im/1
  Convert/1 -> Re/1
  Mult1/1 -> Convert1/1
  Mult/1 -> Convert/1
  Reinterpret/1 -> Mult1/1
  Reinterpret1/1 -> Mult/1
  Slice1/1 -> Reinterpret/1
  Slice/1 -> Reinterpret1/1

== system c960x4096_x14_7_r2013b_frb/p1_scale/SCALE_Re_&_Im_6 ==
  P_S : Inport
  SCALE : Inport  Port=2
  Convert : xbsIndex_r4/Convert  gui_display_data_type=Fixed-point  arith_type="Signed  (2's comp)"  n_bits=8  bin_pt=5  float_type=Single  exp_bits=8  fraction_bits=24  quantization=Truncate  overflow=Wrap  en=off  latency=0  dbl_ovrd=off  pipeline=off  block_type=convert
  Convert1 : xbsIndex_r4/Convert  gui_display_data_type=Fixed-point  arith_type="Signed  (2's comp)"  n_bits=8  bin_pt=5  float_type=Single  exp_bits=8  fraction_bits=24  quantization=Truncate  overflow=Wrap  en=off  latency=0  dbl_ovrd=off  pipeline=off  block_type=convert
  Mult : xbsIndex_r4/Mult  precision=Full  arith_type="Signed  (2's comp)"  n_bits=16  bin_pt=14  quantization=Truncate  overflow=Wrap  en=off  latency=4  dbl_ovrd=off  use_behavioral_HDL=off  opt=Speed  use_embedded=on  optimum_pipeline=off  pipeline=on  use_rpm=on  placement_style=Triangular  block_type=mult
  Mult1 : xbsIndex_r4/Mult  precision=Full  arith_type="Signed  (2's comp)"  n_bits=16  bin_pt=14  quantization=Truncate  overflow=Wrap  en=off  latency=4  dbl_ovrd=off  use_behavioral_HDL=off  opt=Speed  use_embedded=on  optimum_pipeline=off  pipeline=on  use_rpm=on  placement_style=Triangular  block_type=mult
  Reinterpret : xbsIndex_r4/Reinterpret  force_arith_type=on  arith_type="Signed  (2's comp)"  force_bin_pt=on  bin_pt=17  block_type=reinterpret
  Reinterpret1 : xbsIndex_r4/Reinterpret  force_arith_type=on  arith_type="Signed  (2's comp)"  force_bin_pt=on  bin_pt=17  block_type=reinterpret
  Slice : xbsIndex_r4/Slice  nbits=18  boolean_output=off  mode=Upper Bit Location + Width  bit1=0  base1=MSB of Input  bit0=0  base0=LSB of Input  dbl_ovrd=off  block_type=slice
  Slice1 : xbsIndex_r4/Slice  nbits=18  boolean_output=off  mode=Lower Bit Location + Width  bit1=0  base1=MSB of Input  bit0=0  base0=LSB of Input  dbl_ovrd=off  block_type=slice
  Re : Outport
  Im : Outport  Port=2
  wires:
  SCALE/1 -> Mult/2, Mult1/2
  P_S/1 -> Slice1/1, Slice/1
  Convert1/1 -> Im/1
  Convert/1 -> Re/1
  Mult1/1 -> Convert1/1
  Mult/1 -> Convert/1
  Reinterpret/1 -> Mult1/1
  Reinterpret1/1 -> Mult/1
  Slice1/1 -> Reinterpret/1
  Slice/1 -> Reinterpret1/1

== system c960x4096_x14_7_r2013b_frb/p1_scale/SCALE_Re_&_Im_7 ==
  P_S : Inport
  SCALE : Inport  Port=2
  Convert : xbsIndex_r4/Convert  gui_display_data_type=Fixed-point  arith_type="Signed  (2's comp)"  n_bits=8  bin_pt=5  float_type=Single  exp_bits=8  fraction_bits=24  quantization=Truncate  overflow=Wrap  en=off  latency=0  dbl_ovrd=off  pipeline=off  block_type=convert
  Convert1 : xbsIndex_r4/Convert  gui_display_data_type=Fixed-point  arith_type="Signed  (2's comp)"  n_bits=8  bin_pt=5  float_type=Single  exp_bits=8  fraction_bits=24  quantization=Truncate  overflow=Wrap  en=off  latency=0  dbl_ovrd=off  pipeline=off  block_type=convert
  Mult : xbsIndex_r4/Mult  precision=Full  arith_type="Signed  (2's comp)"  n_bits=16  bin_pt=14  quantization=Truncate  overflow=Wrap  en=off  latency=4  dbl_ovrd=off  use_behavioral_HDL=off  opt=Speed  use_embedded=on  optimum_pipeline=off  pipeline=on  use_rpm=on  placement_style=Triangular  block_type=mult
  Mult1 : xbsIndex_r4/Mult  precision=Full  arith_type="Signed  (2's comp)"  n_bits=16  bin_pt=14  quantization=Truncate  overflow=Wrap  en=off  latency=4  dbl_ovrd=off  use_behavioral_HDL=off  opt=Speed  use_embedded=on  optimum_pipeline=off  pipeline=on  use_rpm=on  placement_style=Triangular  block_type=mult
  Reinterpret : xbsIndex_r4/Reinterpret  force_arith_type=on  arith_type="Signed  (2's comp)"  force_bin_pt=on  bin_pt=17  block_type=reinterpret
  Reinterpret1 : xbsIndex_r4/Reinterpret  force_arith_type=on  arith_type="Signed  (2's comp)"  force_bin_pt=on  bin_pt=17  block_type=reinterpret
  Slice : xbsIndex_r4/Slice  nbits=18  boolean_output=off  mode=Upper Bit Location + Width  bit1=0  base1=MSB of Input  bit0=0  base0=LSB of Input  dbl_ovrd=off  block_type=slice
  Slice1 : xbsIndex_r4/Slice  nbits=18  boolean_output=off  mode=Lower Bit Location + Width  bit1=0  base1=MSB of Input  bit0=0  base0=LSB of Input  dbl_ovrd=off  block_type=slice
  Re : Outport
  Im : Outport  Port=2
  wires:
  SCALE/1 -> Mult/2, Mult1/2
  P_S/1 -> Slice1/1, Slice/1
  Convert1/1 -> Im/1
  Convert/1 -> Re/1
  Mult1/1 -> Convert1/1
  Mult/1 -> Convert/1
  Reinterpret/1 -> Mult1/1
  Reinterpret1/1 -> Mult/1
  Slice1/1 -> Reinterpret/1
  Slice/1 -> Reinterpret1/1

== system c960x4096_x14_7_r2013b_frb/spec_tick_gen/edge_detect3 ==
  in : Inport
  Delay : xbsIndex_r4/Delay  rst=off  infoeditControl=Selection of Reset will increase slice count due to use of real FFs and instead of SRLs  en=off  latency=1  dbl_ovrd=off  reg_retiming=off  block_type=delay
      settings: xl_area=[0, 0, 0, 0, 0, 0, 0]
  Inverter : xbsIndex_r4/Inverter  en=off  latency=0  dbl_ovrd=off  block_type=inv
      settings: xl_area=[0, 0, 0, 0, 0, 0, 0]
  edge_op : xbsIndex_r4/Logical  logical_function=AND  inputs=2  en=off  latency=0  precision=Full  arith_type=Unsigned  n_bits=8  bin_pt=2  align_bp=on  dbl_ovrd=off  block_type=logical
      settings: xl_area=[0, 0, 0, 0, 0, 0, 0]
  out : Outport
  wires:
  Inverter/1 -> edge_op/1
  edge_op/1 -> out/1
  in/1 -> Inverter/1, Delay/1
  Delay/1 -> edge_op/2

== system c960x4096_x14_7_r2013b_frb/ssg/SuperSlice ==
  In : Inport
  Slice1 : xbsIndex_r4/Slice  nbits=27  boolean_output=off  mode=Lower Bit Location + Width  bit1=0  base1=MSB of Input  bit0=5  base0=LSB of Input  dbl_ovrd=off  block_type=slice
      settings: infoedit="Extracts a given range of bits from each input sample and presents it at the output.  The output type is ordinarily unsigned with binary point at zero, but can be Boolean when the slice is one bit wide.<P><P>Hardware notes: In hardware this block costs nothing."  block_version=10.1.2
  Slice2 : xbsIndex_r4/Slice  nbits=1  boolean_output=off  mode=Lower Bit Location + Width  bit1=0  base1=MSB of Input  bit0=4  base0=LSB of Input  dbl_ovrd=off  block_type=slice
      settings: infoedit="Extracts a given range of bits from each input sample and presents it at the output.  The output type is ordinarily unsigned with binary point at zero, but can be Boolean when the slice is one bit wide.<P><P>Hardware notes: In hardware this block costs nothing."  block_version=10.1.2
  Slice3 : xbsIndex_r4/Slice  nbits=1  boolean_output=off  mode=Lower Bit Location + Width  bit1=0  base1=MSB of Input  bit0=3  base0=LSB of Input  dbl_ovrd=off  block_type=slice
      settings: infoedit="Extracts a given range of bits from each input sample and presents it at the output.  The output type is ordinarily unsigned with binary point at zero, but can be Boolean when the slice is one bit wide.<P><P>Hardware notes: In hardware this block costs nothing."  block_version=10.1.2
  Slice4 : xbsIndex_r4/Slice  nbits=1  boolean_output=off  mode=Lower Bit Location + Width  bit1=0  base1=MSB of Input  bit0=2  base0=LSB of Input  dbl_ovrd=off  block_type=slice
      settings: infoedit="Extracts a given range of bits from each input sample and presents it at the output.  The output type is ordinarily unsigned with binary point at zero, but can be Boolean when the slice is one bit wide.<P><P>Hardware notes: In hardware this block costs nothing."  block_version=10.1.2
  Slice5 : xbsIndex_r4/Slice  nbits=1  boolean_output=off  mode=Lower Bit Location + Width  bit1=0  base1=MSB of Input  bit0=1  base0=LSB of Input  dbl_ovrd=off  block_type=slice
  Slice6 : xbsIndex_r4/Slice  nbits=1  boolean_output=off  mode=Lower Bit Location + Width  bit1=0  base1=MSB of Input  bit0=0  base0=LSB of Input  dbl_ovrd=off  block_type=slice
  "[31:5]" : Outport
  "[4]" : Outport  Port=2
  "[3]" : Outport  Port=3
  "[2]" : Outport  Port=4
  "[1]" : Outport  Port=5
  "[0]" : Outport  Port=6
  wires:
  Slice6/1 -> "[0]"/1
  Slice5/1 -> "[1]"/1
  Slice4/1 -> "[2]"/1
  Slice3/1 -> "[3]"/1
  Slice2/1 -> "[4]"/1
  Slice1/1 -> "[31:5]"/1
  In/1 -> Slice1/1, Slice2/1, Slice3/1, Slice4/1, Slice5/1, Slice6/1

== system c960x4096_x14_7_r2013b_frb/ssg/bus_create1 ==
  in1 : Inport
  in2 : Inport  Port=2
  in3 : Inport  Port=3
  in4 : Inport  Port=4
  concatenate : xbsIndex_r4/Concat  num_inputs=4  dbl_ovrd=off  block_type=concat
  reinterpret{1..4} (4 alike) : xbsIndex_r4/Reinterpret  force_arith_type=on  arith_type=Unsigned  force_bin_pt=on  bin_pt=0  block_type=reinterpret
      reinterpret1 settings: infoedit="Changes signal type without altering the binary representation.   You can changed the signal between signed and unsigned, and relocate the binary point.<br><br>Hardware notes: In hardware this block costs nothing.<br><br>Example:  Suppose the input is 6 bits wide, signed, with 2 fractional bits, and the output is forced to unsigned with 0 fractional bits.  Then an input of -2.0 (1110.00 in binary 2's complement) becomes an output of 56 (111000 in binary)."
      reinterpret2 settings: infoedit="Changes signal type without altering the binary representation.   You can changed the signal between signed and unsigned, and relocate the binary point.<br><br>Hardware notes: In hardware this block costs nothing.<br><br>Example:  Suppose the input is 6 bits wide, signed, with 2 fractional bits, and the output is forced to unsigned with 0 fractional bits.  Then an input of -2.0 (1110.00 in binary 2's complement) becomes an output of 56 (111000 in binary)."
  bus_out : Outport
  wires:
  reinterpret4/1 -> concatenate/4
  in4/1 -> reinterpret4/1
  reinterpret3/1 -> concatenate/3
  in3/1 -> reinterpret3/1
  reinterpret2/1 -> concatenate/2
  in2/1 -> reinterpret2/1
  reinterpret1/1 -> concatenate/1
  in1/1 -> reinterpret1/1
  concatenate/1 -> bus_out/1

== system c960x4096_x14_7_r2013b_frb/ssg/bus_create2 ==
  in1 : Inport
  in2 : Inport  Port=2
  in3 : Inport  Port=3
  in4 : Inport  Port=4
  concatenate : xbsIndex_r4/Concat  num_inputs=4  dbl_ovrd=off  block_type=concat
  reinterpret{1..4} (4 alike) : xbsIndex_r4/Reinterpret  force_arith_type=on  arith_type=Unsigned  force_bin_pt=on  bin_pt=0  block_type=reinterpret
      reinterpret1 settings: infoedit="Changes signal type without altering the binary representation.   You can changed the signal between signed and unsigned, and relocate the binary point.<br><br>Hardware notes: In hardware this block costs nothing.<br><br>Example:  Suppose the input is 6 bits wide, signed, with 2 fractional bits, and the output is forced to unsigned with 0 fractional bits.  Then an input of -2.0 (1110.00 in binary 2's complement) becomes an output of 56 (111000 in binary)."
      reinterpret2 settings: infoedit="Changes signal type without altering the binary representation.   You can changed the signal between signed and unsigned, and relocate the binary point.<br><br>Hardware notes: In hardware this block costs nothing.<br><br>Example:  Suppose the input is 6 bits wide, signed, with 2 fractional bits, and the output is forced to unsigned with 0 fractional bits.  Then an input of -2.0 (1110.00 in binary 2's complement) becomes an output of 56 (111000 in binary)."
  bus_out : Outport
  wires:
  reinterpret4/1 -> concatenate/4
  in4/1 -> reinterpret4/1
  reinterpret3/1 -> concatenate/3
  in3/1 -> reinterpret3/1
  reinterpret2/1 -> concatenate/2
  in2/1 -> reinterpret2/1
  reinterpret1/1 -> concatenate/1
  in1/1 -> reinterpret1/1
  concatenate/1 -> bus_out/1
